simulink model "cuircuitB"  (R2022b)
settings: Solver=VariableStepAuto  StartTime=0.0  StopTime=100  RelTol=1e-3
libraries: fuzblock x1
settings Model: Creator=andre  LastModifiedBy=Paulo Cortesão

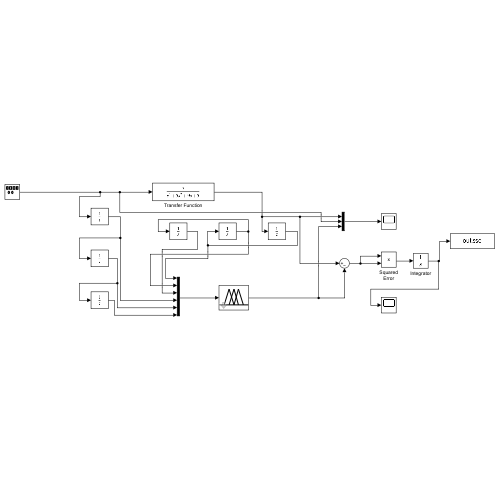
[thumbnail: Simulink's stored preview of the top-level diagram]
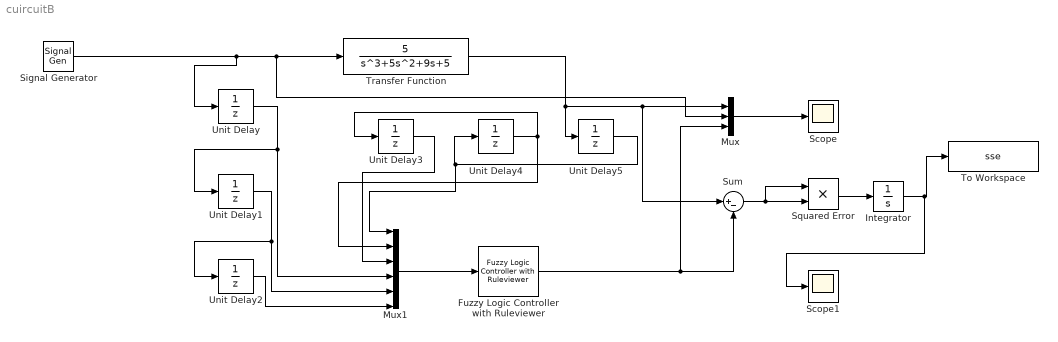
== system cuircuitB ==
  Fuzzy Logic Controller with Ruleviewer : fuzblock/Fuzzy Logic  Controller  with Ruleviewer  fismatrix=fis_test  Ts=0.125
  Integrator : Integrator
  Mux : Mux  Inputs=3
  Mux1 : Mux  Inputs=6
  Scope : Scope
  Scope1 : Scope
  Signal Generator : SignalGenerator  WaveForm=square  Amplitude=-1  Frequency=0.10  Units=rad/sec
  Squared Error : Product
  Sum : Sum  Inputs=|+-
  To Workspace : ToWorkspace  VariableName=sse  SaveFormat=Timeseries  SampleTime=-1
  Transfer Function : TransferFcn  Numerator=[5]  Denominator=[1 5 9 5]
  Unit Delay{,1..5} (6 alike) : UnitDelay  SampleTime=-1  HasFrameUpgradeWarning=on
  wires:
  Signal Generator/1 -> Unit Delay/1, Mux/2, Transfer Function/1
  Unit Delay/1 -> Mux1/4, Unit Delay1/1
  Unit Delay1/1 -> Mux1/5, Unit Delay2/1
  Unit Delay2/1 -> Mux1/6
  Unit Delay4/1 -> Mux1/2, Unit Delay3/1
  Unit Delay5/1 -> Mux1/1, Unit Delay4/1
  Unit Delay3/1 -> Mux1/3
  Mux1/1 -> Fuzzy Logic Controller with Ruleviewer/1
  Fuzzy Logic Controller with Ruleviewer/1 -> Sum/2, Mux/3
  Transfer Function/1 -> Unit Delay5/1, Sum/1, Mux/1
  Mux/1 -> Scope/1
  Sum/1 -> Squared Error/1, Squared Error/2
  Squared Error/1 -> Integrator/1
  Integrator/1 -> Scope1/1, To Workspace/1
